simulink model "UNICO"  (R2023b)
settings: Solver=FixedStepDiscrete  StartTime=0.0  StopTime=inf  FixedStep=Control.DT  RelTol=1e-3
undefined symbols (not defined in the file): Control
libraries: cstblocks x5, simulink x2
(part 3 of 3)

== matlab function UNICO/PI CONTROLLER/Initialize integral term ==
  data: checkDelay input; check output; PI_int input; PI_int output; wg input; WindSpeed input; Architecture_Selector input; Darrieus_Selector input; Params input; propTerm input
function [check,PI_int] = fcn(checkDelay, PI_int, wg, WindSpeed, Architecture_Selector, Darrieus_Selector, Params, propTerm)
% Load R struct variables
R       = Params(1);  % Rotor radius                       [m]
v_rt    = Params(2);  % Rated power wind speed             [m/s]
Tq_rated = Params(3); % Rated torque                       [Nm]
w_rt    = Params(5);  % Rated generator speed              [rad/s]
w_min   = Params(9);  % Minimum generator speed            [rad/s]
r2      = Params(10); % Region 2 control mode  {0: optimum tsr tracking; 1: kw^2 torque law}
KSwitch = Params(11); % Region 2 K- switch
Rgn2K = Params(12);   % user defined K value
SpdSwitch = Params(13); %generator speed for switch between region 2 and 2 1/2
w_minSwitch = Params(14); % Switch between region 1.5 and 2 [rad/s]
TSR_opt = Params(15);  % Optimum TSR                             [-]
Cpmax   = Params(16); % max cp value                             [-]
rho     = Params(22);  % Air density                             [kg/m^3]
Bld_Height = Params(24); %Blades Height (VAWT ONLY)              [m]   
Rot_area= Params(28); % Rotor Area (VAWT Eggbeater Type ONLY) [m^2]

% ===========================================
% PRIMA: Controlla se siamo in Regione 3
% (questo deve essere fatto INDIPENDENTEMENTE da r2)
% ===========================================
if WindSpeed > v_rt
    % REGIONE 3
    check = 3;
    
    % Inizializza l'integratore quando entriamo in Regione 3
    if checkDelay ~= 3
        % Stiamo entrando in Regione 3 da un'altra regione
        % Inizializza l'integratore per dare Torque = Torque_rated
        PI_int = Tq_rated - propTerm;
    end
    % Se checkDelay == 3, siamo già in Regione 3, non toccare l'integratore

% ===========================================
% ALTRIMENTI: Siamo in Regione 2 o inferiore
% ===========================================
else
    if r2 == 1
        % Modalità k-omega^2
        w1  = SpdSwitch;
        if KSwitch == 1
            K = Rgn2K;
        else
            if Architecture_Selector == 1
                K   = 0.5*rho*pi*R^5*Cpmax/TSR_opt^3;  % K coefficient for HAWT
            else
                if Darrieus_Selector == 1
                    K   = rho*R^4*Bld_Height*Cpmax/TSR_opt^3;  % K coefficient for VAWT - H Type
                else 
                    K = 0.5*rho*Rot_area*R^3*Cpmax/TSR_opt^3;  % K coefficient for VAWT - Eggbeater Type
                end
            end
        end
        
        if (wg < w1) && (WindSpeed <= v_rt)
            % region 2. Store idx to check at following time step
            if wg < w_minSwitch
                % Region 1.5 We have to evaluate if we need to initialize the
                % integral term
                check = 0;
                if checkDelay == 2 % we are coming from region 2, initialize to the k-w^2 value at wg = w1
                    Tg1 = K*wg^2; % torque value from k-w^2 law
                    PI_int = (Tg1)-propTerm;  %initialize integral term
                elseif checkDelay == 0
                    % we were already in Region 1.5
                    % do not initialize Integral term
                end
            else
                % we are in region 2
                check = 2; 
            end
        elseif (wg < w_rt) && (WindSpeed <= v_rt) % we are in 2 1/2
            % region 2 1/2. We have to evaluate if we need to initialize the
            % integral term
            check = 1;
            if checkDelay == 2 % we are coming from region 2, initialize to the k-w^2 value at wg = w1
                Tg1 = K*wg^2; % torque value from k-w^2 law
                PI_int = (Tg1)-propTerm;  %initialize integral term
            elseif checkDelay == 3
                % when coming from region 3 do not modify integral term, we are
                % already using PI controller
            else
                % do not modify integral term, checkDelay = 1 -> PI controller
                % already running. 
            end
        else
            % Questo caso non dovrebbe mai verificarsi perché WindSpeed <= v_rt
            % ma per sicurezza
            check = 0;
        end
    else
        % r2 == 0: TSR tracking con PI controller
        % Non modificare PI_int, il controller PI gestisce tutto
        check = 0;
    end
end
